simulink model "QuyDaoLapTrinh_2020a"  (R2020a)
settings: Solver=VariableStepAuto  StartTime=0.0  StopTime=10.0  RelTol=1e-3
settings Model: Creator=Hp  LastModifiedBy=Hp
settings DebuggingCC: SFMachineParentedDataDiag=error

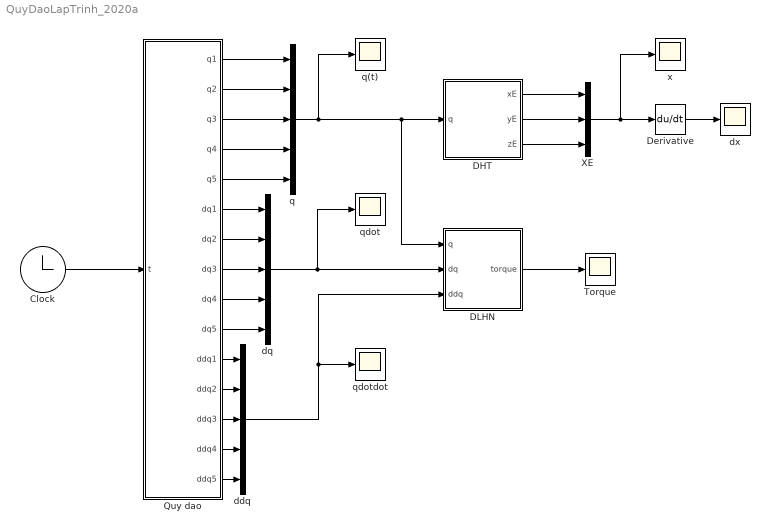
== system QuyDaoLapTrinh_2020a ==
  Clock : Clock
  DHT : MATLAB Function  TreatAsAtomicUnit=on
  DLHN : MATLAB Function  TreatAsAtomicUnit=on
  Derivative : Derivative
  "Quy dao " : MATLAB Function  TreatAsAtomicUnit=on
  Torque : Scope
  XE : Mux  Inputs=3
  ddq : Mux  Inputs=5
  dq : Mux  Inputs=5
  dx : Scope
  q : Mux  Inputs=5
  q(t) : Scope
  qdot : Scope
  qdotdot : Scope
  x : Scope
  wires:
  Clock/1 -> "Quy dao "/1(t)
  "Quy dao "/1(q1) -> q/1
  "Quy dao "/2(q2) -> q/2
  "Quy dao "/3(q3) -> q/3
  "Quy dao "/4(q4) -> q/4
  "Quy dao "/5(q5) -> q/5
  "Quy dao "/6(dq1) -> dq/1
  "Quy dao "/7(dq2) -> dq/2
  "Quy dao "/8(dq3) -> dq/3
  "Quy dao "/9(dq4) -> dq/4
  "Quy dao "/10(dq5) -> dq/5
  "Quy dao "/11(ddq1) -> ddq/1
  "Quy dao "/12(ddq2) -> ddq/2
  "Quy dao "/13(ddq3) -> ddq/3
  "Quy dao "/14(ddq4) -> ddq/4
  "Quy dao "/15(ddq5) -> ddq/5
  q/1 -> q(t)/1, DHT/1(q), DLHN/1(q)
  DHT/1(xE) -> XE/1
  DHT/2(yE) -> XE/2
  DHT/3(zE) -> XE/3
  XE/1 -> Derivative/1, x/1
  DLHN/1(torque) -> Torque/1
  Derivative/1 -> dx/1
  dq/1 -> DLHN/2(dq), qdot/1
  ddq/1 -> qdotdot/1, DLHN/3(ddq)

== matlab function QuyDaoLapTrinh_2020a/DLHN ==
  data: q input; torque output; dq input; ddq input
function torque = fcn(q, dq, ddq)
L1=2; % m
L2=2;
a2=1;
L3=1.5;
L4=1;
L5=0.75;

m2=2;
m3=1;
m4=0.75;
m5=0.5;

I2x=10^(-4);
I2y=10^(-4);
I2z=10^(-4);

I3x=10^(-4);
I3y=10^(-4);
I3z=10^(-4);

I4x=10^(-4);
I4y=10^(-4);
I4z=10^(-4);

I5x=10^(-4);
I5y=10^(-4);
I5z=10^(-4);
%Ma tran M
M=zeros(5,5);
M(1,1)= m2 + m3 + m4 + m5;
M(1,2)= -((m5 * (2 * L4 + L5) + m4 * L4) * cos(q(4)) + (2 * a2 * (m3 + m4 + m5))) * sin(q(2)) / 0.2e1;
M(1,3)= 0;
M(1,4)= -sin(q(4)) * cos(q(2)) * ((m4 + 2 * m5) * L4 + m5 * L5) / 0.2e1;
M(1,5)= 0;

M(2,1)= -((m5 * (2 * L4 + L5) + m4 * L4) * cos(q(4)) + (2 * a2 * (m3 + m4 + m5))) * sin(q(2)) / 0.2e1;
M(2,2)= ((-4 * I5x + 4 * I5y) * cos(q(5)) ^ 2 + 0.4e1 * (L4 + L5 / 0.2e1) ^ 2 * m5 + m4 * L4 ^ 2 - (4 * I4x) + (4 * I4y) + (4 * I5x) - (4 * I5z)) * cos(q(4)) ^ 2 / 0.4e1 + (m5 * (0.2e1 * L4 + L5) + m4 * L4) * a2 * cos(q(4)) + ((4 * m3) + 0.4e1 * m4 + 0.4e1 * m5) * a2 ^ 2 / 0.4e1 + I3z + I4x + I5z + I2z;
M(2,3)= 0;
M(2,4)= sin(q(5)) * cos(q(5)) * cos(q(4)) * (I5x - I5y);
M(2,5)= -sin(q(4)) * I5z;

M(3,1)= 0;
M(3,2)= 0;
M(3,3)= m3 + m4 + m5;
M(3,4)= -((m4 + 2 * m5) * L4 + m5 * L5) * cos(q(4)) / 0.2e1;
M(3,5)= 0;

M(4,1)= -sin(q(4)) * cos(q(2)) * ((m4 + 2 * m5) * L4 + m5 * L5) / 0.2e1;
M(4,2)= sin(q(5)) * cos(q(5)) * cos(q(4)) * (I5x - I5y);
M(4,3)= -((m4 + 2 * m5) * L4 + m5 * L5) * cos(q(4)) / 0.2e1;
M(4,4)= m4 * L4 ^ 2 / 0.4e1 + I4z + (I5x - I5y) * cos(q(5)) ^ 2 + (0.2e1 * L4 + L5) ^ 2 * m5 / 0.4e1 + I5y;
M(4,5)= 0;

M(5,1)= 0;
M(5,2)= -sin(q(4)) * I5z;
M(5,3)= 0;
M(5,4)= 0;
M(5,5)= I5z

%Ma tran C
C=zeros(5,5);
C(1,1)= 0;
C(1,2)= -((m5 * (2 * L4 + L5) + m4 * L4) * cos(q(4)) + (2 * a2 * (m3 + m4 + m5))) * cos(q(2)) * dq(2) / 0.2e1 + sin(q(4)) * (m5 * (2 * L4 + L5) + m4 * L4) * sin(q(2)) * dq(4) / 0.2e1;
C(1,3)= 0;
C(1,4)= -(dq(4) * cos(q(2)) * cos(q(4)) - dq(2) * sin(q(2)) * sin(q(4))) * ((m4 + 2 * m5) * L4 + m5 * L5) / 0.2e1;
C(1,5)= 0;

C(2,1)= -((m5 * (2 * L4 + L5) + m4 * L4) * cos(q(4)) + (2 * a2 * (m3 + m4 + m5))) * cos(q(2)) * dq(2) / 0.4e1 + sin(q(4)) * (m5 * (2 * L4 + L5) + m4 * L4) * sin(q(2)) * dq(4) / 0.4e1;
C(2,2)= 0.2e1 * dq(5) * cos(q(5)) * sin(q(5)) * (I5x - I5y) * cos(q(4)) ^ 2 + (-0.2e1 * dq(4) * ((-0.4e1 * I5x + 0.4e1 * I5y) * cos(q(5)) ^ 2 + 0.4e1 * (L4 + L5 / 0.2e1) ^ 2 * m5 + m4 * L4 ^ 2 - (4 * I4x) + (4 * I4y) + 0.4e1 * I5x - (4 * I5z)) * sin(q(4)) + cos(q(2)) * (m5 * (0.2e1 * L4 + L5) + m4 * L4) * dq(1)) * cos(q(4)) / 0.4e1 - a2 * (dq(4) * (m5 * (0.2e1 * L4 + L5) + m4 * L4) * sin(q(4)) - dq(1) * cos(q(2)) * (m3 + m4 + m5) / 0.2e1);
C(2,3)= 0;
C(2,4)=  (-0.4e1 * (I5x - I5y) * cos(q(5)) * sin(q(5)) * dq(4) - ((m4 + 2 * m5) * L4 + m5 * L5) * dq(1) * sin(q(2))) * sin(q(4)) / 0.4e1 + 0.2e1 * (I5x - I5y) * cos(q(4)) * (cos(q(5)) ^ 2 - 0.1e1 / 0.2e1) * dq(5);
C(2,5)= -I5z * cos(q(4)) * dq(4);

C(3,1)= 0;
C(3,2)= 0;
C(3,3)= 0;
C(3,4)=((m4 + 2 * m5) * L4 + m5 * L5) * sin(q(4)) * dq(4) / 0.2e1;
C(3,5)= 0;

C(4,1)= -(dq(4) * cos(q(2)) * cos(q(4)) - dq(2) * sin(q(2)) * sin(q(4))) * ((m4 + 2 * m5) * L4 + m5 * L5) / 0.4e1;
C(4,2)= (((-4 * I5x + 4 * I5y) * cos(q(5)) ^ 2 + ((m4 + 4 * m5) * L4 ^ 2) + (4 * L4 * L5 * m5) + (L5 ^ 2 * m5) + (4 * I5x) - (4 * I5z) - (4 * I4x) + (4 * I4y)) * dq(2) * cos(q(4)) - 0.2e1 * (I5x - I5y) * cos(q(5)) * sin(q(5)) * dq(4) - (dq(1) * sin(q(2)) - 0.2e1 * dq(2) * a2) * ((m4 + 2 * m5) * L4 + m5 * L5)) * sin(q(4)) / 0.4e1 + 0.2e1 * cos(q(4)) * dq(5) * ((I5x - I5y) * cos(q(5)) ^ 2 - I5x / 0.2e1 + I5y / 0.2e1 + I5z / 0.4e1);
C(4,3)= ((m4 + 2 * m5) * L4 + m5 * L5) * sin(q(4)) * dq(4) / 0.4e1;
C(4,4)= (0.2e1 * dq(2) * sin(q(5)) * (I5x - I5y) * cos(q(5)) - (((m4 + 2 * m5) * L4 + m5 * L5) * dq(3))) * sin(q(4)) / 0.4e1 - 0.2e1 * (I5x - I5y) * cos(q(5)) * sin(q(5)) * dq(5) + cos(q(4)) * cos(q(2)) * ((m4 + 2 * m5) * L4 + m5 * L5) * dq(1) / 0.4e1;
C(4,5)= I5z * cos(q(4)) * dq(2) / 0.2e1;

C(5,1)= 0;
C(5,2)= -cos(q(4)) * (dq(4) * (I5x - I5y) * cos(q(5)) ^ 2 + sin(q(5)) * dq(2) * cos(q(4)) * (I5x - I5y) * cos(q(5)) - dq(4) * (I5x - I5y - (2 * I5z)) / 0.2e1);
C(5,3)= 0;
C(5,4)= -(I5x - I5y) * (dq(2) * (cos(q(5)) ^ 2 - 0.1e1 / 0.2e1) * cos(q(4)) - cos(q(5)) * sin(q(5)) * dq(4));
C(5,5)= 0;

%Ma tran G
G=zeros(5,1);
G(1,1)= 0;
G(2,1)= 0;
G(3,1)= 10*(m3 + m4);
G(4,1)= -5*m4*L4*cos(q(4));
G(5,1)= 0;

torque = M*ddq + C*dq + G;

== matlab function QuyDaoLapTrinh_2020a/Quy dao  ==
  data: t input; q1 output; q2 output; q3 output; q4 output; q5 output; dq1 output; dq2 output; dq3 output; dq4 output; dq5 output; ddq1 output; ddq2 output; ddq3 output; ddq4 output; ddq5 output
function [q1,q2,q3,q4,q5,dq1,dq2,dq3,dq4,dq5,ddq1,ddq2,ddq3,ddq4,ddq5] = fcn(t)
q1= 0.2e1 + 0.9e1 / 0.100e3 * t ^ 2 - 0.3e1 / 0.500e3 * t ^ 3;
q2= pi / 0.3e1 + pi * t ^ 2 / 0.200e3 - pi * t ^ 3 / 0.3000e4;
q3= 0.2e1 + 0.3e1 / 0.100e3 * t ^ 2 - t ^ 3 / 0.500e3;
q4= pi / 0.6e1 + pi * t ^ 2 / 0.400e3 - pi * t ^ 3 / 0.6000e4;
q5=0;

dq1= 0.9e1 / 0.50e2 * t - 0.9e1 / 0.500e3 * t ^ 2;
dq2= pi * t / 0.100e3 - pi * t ^ 2 / 0.1000e4;
dq3= 0.3e1 / 0.50e2 * t - 0.3e1 / 0.500e3 * t ^ 2;
dq4= pi * t / 0.200e3 - pi * t ^ 2 / 0.2000e4;
dq5=0;

ddq1=0.18-0.036*t;
ddq2=(pi/100)-(pi/500)*t;
ddq3=0.06-0.012*t;
ddq4=(pi/200)-(pi/1000)*t;
ddq5=0;
end

== matlab function QuyDaoLapTrinh_2020a/DHT ==
  data: q input; xE output; yE output; zE output
function [xE,yE,zE] = fcn(q)
%Khai bao thong so 
L1=2;
L2=1;
a2=1;
L3=1.5;
L4=1;
L5=0.75;
%Phuong trinh dong hoc thuan
xE=((L4 + L5) * cos(q(4)) + a2) * cos(q(2)) + q(1);
yE=sin(q(2)) * ((L4 + L5) * cos(q(4)) + a2);
zE=(-L4 - L5) * sin(q(4)) + q(3) + L2;
end
